simulink model "CondenserMic"  (R2024a)
settings: Solver=daessc  StartTime=0.0  StopTime=T  MaxStep=1e-4  RelTol=1e-3
PreLoadFcn:
  | f_in = 1000;
model workspace (MAT data in the model file):
  A = Simulink.Parameter
  A.Value = Simulink.data.Expression
  A.Value.ExpressionString = "pi*r^2"
  A.Complexity = 'real'
  A.Dimensions = -1
  A.Description = 'diaphragm area'
  A.DataType = 'auto'
  A.DocUnits = 'm^2'
  A_bp = Simulink.Parameter
  A_bp.Value = Simulink.data.Expression
  A_bp.Value.ExpressionString = "pi*r_bp^2"
  A_bp.Complexity = 'real'
  A_bp.Dimensions = -1
  A_bp.DataType = 'auto'
  A_bp.DocUnits = 'm^2'
  Ceo = Simulink.Parameter
  Ceo.Value = 1.85e-11
  Ceo.Complexity = 'real'
  Ceo.Dimensions = [1 1]
  Ceo.Description = 'microphone open circuit capacitance'
  Ceo.DataType = 'auto'
  Ceo.DocUnits = 'F'
  N_hole = Simulink.Parameter
  N_hole.Value = 6
  N_hole.Complexity = 'real'
  N_hole.Dimensions = [1 1]
  N_hole.Description = 'number of holes on back plate'
  N_hole.DataType = 'auto'
  N_vent = Simulink.Parameter
  N_vent.Value = 6
  N_vent.Complexity = 'real'
  N_vent.Dimensions = [1 1]
  N_vent.Description = 'number of rear vent'
  N_vent.DataType = 'auto'
  T = Simulink.Parameter
  T.Value = 5
  T.Complexity = 'real'
  T.Dimensions = [1 1]
  T.Description = 'simulation time '
  T.DataType = 'auto'
  Vb = Simulink.Parameter
  Vb.Value = 1.264e-07
  Vb.Complexity = 'real'
  Vb.Dimensions = [1 1]
  Vb.Description = 'rear cavity volume'
  Vb.DataType = 'auto'
  Vb.DocUnits = 'm^3'
  c = Simulink.Parameter
  c.Value = 343
  c.Complexity = 'real'
  c.Dimensions = [1 1]
  c.Description = 'sound speed in air'
  c.DataType = 'auto'
  c.DocUnits = 'm/s'
  d1 = Simulink.Parameter
  d1.Value = 0.002032
  d1.Complexity = 'real'
  d1.Dimensions = [1 1]
  d1.Description = 'Radius of the circle intersecting the holes'
  d1.DataType = 'auto'
  d1.DocUnits = 'm'
  dt = Simulink.Parameter
  dt.Value = 2.08333333333e-05
  dt.Complexity = 'real'
  dt.Dimensions = [1 1]
  dt.Description = 'sample time'
  dt.DataType = 'auto'
  eps0 = Simulink.Parameter
  eps0.Value = 8.85e-12
  eps0.Complexity = 'real'
  eps0.Dimensions = [1 1]
  eps0.Description = 'permittivity in vaicuum'
  eps0.DataType = 'auto'
  eps0.DocUnits = 'F/m'
  h_gap = Simulink.Parameter
  h_gap.Value = 2.077e-05
  h_gap.Complexity = 'real'
  h_gap.Dimensions = [1 1]
  h_gap.Description = 'air gap thickness '
  h_gap.DataType = 'auto'
  h_gap.DocUnits = 'm'
  h_hole = Simulink.Parameter
  h_hole.Value = 0.000843
  h_hole.Complexity = 'real'
  h_hole.Dimensions = [1 1]
  h_hole.Description = 'back plate holes depth (thickness)'
  h_hole.DataType = 'auto'
  h_hole.DocUnits = 'm'
  h_slot = Simulink.Parameter
  h_slot.Value = 0.0003048
  h_slot.Complexity = 'real'
  h_slot.Dimensions = [1 1]
  h_slot.Description = 'slot depth (thickness)'
  h_slot.DataType = 'auto'
  h_slot.DocUnits = 'm'
  h_vent = Simulink.Parameter
  h_vent.Value = 0.0015
  h_vent.Complexity = 'real'
  h_vent.Dimensions = [1 1]
  h_vent.Description = 'rear vent depth (thickness)'
  h_vent.DataType = 'auto'
  h_vent.DocUnits = 'm'
  l_slot = Simulink.Parameter
  l_slot.Value = Simulink.data.Expression
  l_slot.Value.ExpressionString = "2*pi*r"
  l_slot.Complexity = 'real'
  l_slot.Dimensions = -1
  l_slot.DataType = 'auto'
  l_slot.DocUnits = 'm'
  l_vent = Simulink.Parameter
  l_vent.Value = 0.00034
  l_vent.Complexity = 'real'
  l_vent.Dimensions = [1 1]
  l_vent.Description = 'rear vent length'
  l_vent.DataType = 'auto'
  l_vent.DocUnits = 'm'
  r = Simulink.Parameter
  r.Value = 0.00445
  r.Complexity = 'real'
  r.Dimensions = [1 1]
  r.Description = 'diaphragm radius'
  r.DataType = 'auto'
  r.DocUnits = 'm'
  r_bp = Simulink.Parameter
  r_bp.Value = 0.00361
  r_bp.Complexity = 'real'
  r_bp.Dimensions = [1 1]
  r_bp.Description = 'back plate radius'
  r_bp.DataType = 'auto'
  r_bp.DocUnits = 'm'
  r_hole = Simulink.Parameter
  r_hole.Value = 0.000508
  r_hole.Complexity = 'real'
  r_hole.Dimensions = [1 1]
  r_hole.Description = 'back plate holes radius'
  r_hole.DataType = 'auto'
  r_hole.DocUnits = 'm'
  rho = Simulink.Parameter
  rho.Value = 1.21
  rho.Complexity = 'real'
  rho.Dimensions = [1 1]
  rho.Description = 'air density'
  rho.DataType = 'auto'
  rho.DocUnits = 'kg/m^3'
  w_slot = Simulink.Parameter
  w_slot.Value = 0.000838
  w_slot.Complexity = 'real'
  w_slot.Dimensions = [1 1]
  w_slot.Description = 'slot width'
  w_slot.DataType = 'auto'
  w_slot.DocUnits = 'm'
  w_vent = Simulink.Parameter
  w_vent.Value = 1.1e-05
  w_vent.Complexity = 'real'
  w_vent.Dimensions = [1 1]
  w_vent.Description = 'rear vent width'
  w_vent.DataType = 'auto'
  w_vent.DocUnits = 'm'
libraries: fl_lib x11, acoustic_lib x7, nesl_utility x3, ee_lib x1
settings Model: Creator=andychen  LastModifiedBy=jibrahim
settings DataIOCC: OutputOption=SpecifiedOutputTimes  OutputTimes=0:dt:T  Refine=0:5e-5:10

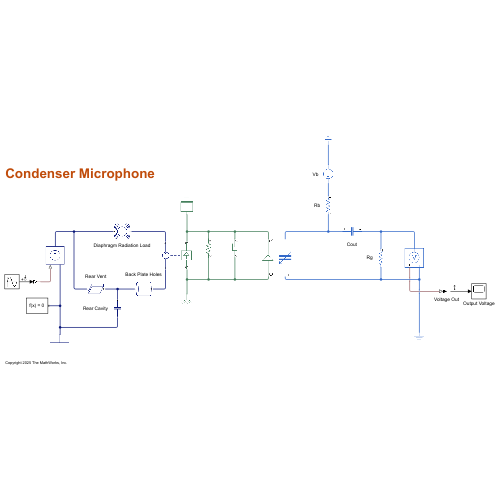
[thumbnail: Simulink's stored preview of the top-level diagram]
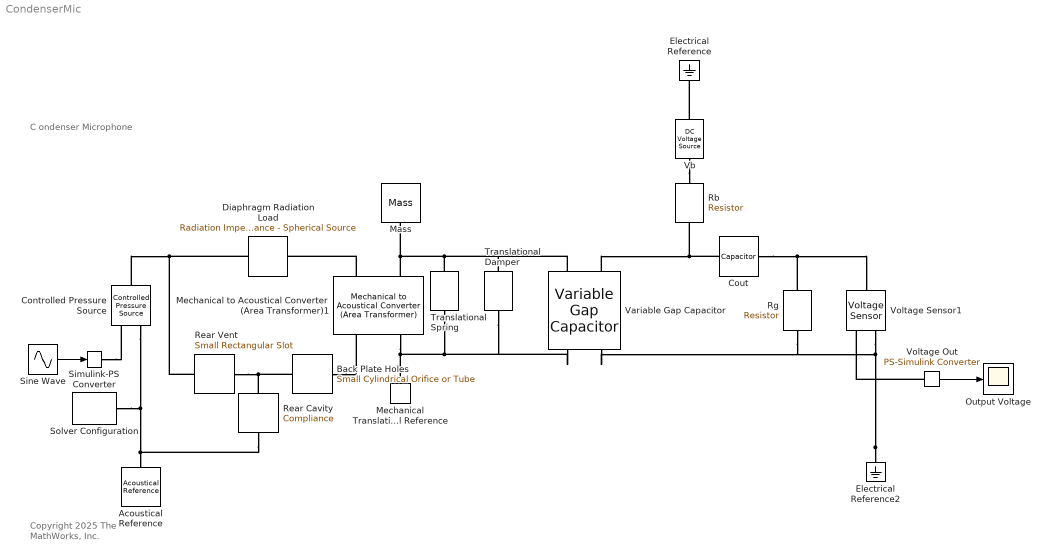
== system CondenserMic ==
  note: C ondenser Microphone
  note: Copyright 2025 The MathWorks, Inc.
  Acoustical Reference : acoustic_lib/Acoustical Elements/Acoustical Reference
      settings: SourceProductName=Acoustic  InternalSimscapePortConfiguration="{\"Bottom\":[],\"Left\":[{\"id\":\"pp\",\"label\":\"\",\"type\":\"acoustic.acoustic\"}],\"Right\":[],\"Top\":[]}"
  Back Plate Holes : acoustic_lib/Applications/Tubes and Horns/Small Cylindrical Orifice or Tube  l=h_hole m  r=r_hole m  N=N_hole
      settings: SourceProductName=Acoustic  InternalSimscapePortConfiguration="{\"Bottom\":[],\"Left\":[{\"id\":\"pa\",\"label\":\"+\",\"type\":\"acoustic.acoustic\"}],\"Right\":[{\"id\":\"na\",\"label\":\"-\",\"type\":\"acoustic.acoustic\"}],\"Top\":[]}"
  Controlled Pressure Source : acoustic_lib/Acoustical Sources/Controlled Pressure Source
      settings: SourceProductName=Acoustic  InternalSimscapePortConfiguration="{\"Bottom\":[],\"Left\":[{\"id\":\"pp\",\"label\":\"\",\"type\":\"acoustic.acoustic\"}],\"Right\":[{\"id\":\"pT\",\"label\":\"\",\"type\":\"input\"},{\"id\":\"nn\",\"label\":\"\",\"type\":\"acoustic.acoustic\"}],\"Top\":[]}"
  Cout : fl_lib/Electrical/Electrical Elements/Capacitor  c=1e-12 F  r=1e-6 Ohm  g=0 1/Ohm  i_specify=off  i_priority=None  i=0 A  i_nominal_specify=off  i_nominal_value=1  i_nominal_unit=A  v_specify=off  v_priority=None  v=0 V  v_nominal_specify=off  v_nominal_value=1  v_nominal_unit=V  vc_specify=off  vc_priority=High  vc=0 V  vc_nominal_specify=off  vc_nominal_value=1  vc_nominal_unit=V
  Diaphragm Radiation Load : acoustic_lib/Radiation Impedance/Radiation Impedance - Spherical Source  r=r m
      settings: SourceProductName=Acoustic  InternalSimscapePortConfiguration="{\"Bottom\":[],\"Left\":[{\"id\":\"pa\",\"label\":\"+\",\"type\":\"acoustic.acoustic\"}],\"Right\":[{\"id\":\"na\",\"label\":\"-\",\"type\":\"acoustic.acoustic\"}],\"Top\":[]}"
  Electrical Reference : fl_lib/Electrical/Electrical Elements/Electrical Reference
  Electrical Reference2 : fl_lib/Electrical/Electrical Elements/Electrical Reference
  Mass : fl_lib/Mechanical/Translational Elements/Mass  mass=9.22e-7 kg  num_ports=foundation.enum.numPorts2.one  v_specify=off  v_priority=High  v=0 m/s  v_nominal_specify=off  v_nominal_value=1  v_nominal_unit=m/s  f_specify=off  f_priority=None  f=0 N  f_nominal_specify=off  f_nominal_value=1  f_nominal_unit=N
  Mechanical Translational Reference : fl_lib/Mechanical/Translational Elements/Mechanical Translational Reference
  Mechanical to Acoustical Converter (Area Transformer)1 : acoustic_lib/Transformers/Mechanical to Acoustical Converter (Area Transformer)  Sd=A m^2  u_specify=off  u_priority=None  u=0 m^3/s  u_nominal_specify=off  u_nominal_value=1  u_nominal_unit=m^3/s  p_specify=off  p_priority=None  p=0 Pa  p_nominal_specify=off  p_nominal_value=1  p_nominal_unit=Pa  f_specify=off  f_priority=None  f=0 N  f_nominal_specify=off  f_nominal_value=1  f_nominal_unit=N  v_specify=off  v_priority=None  v=0 m/s  v_nominal_specify=off  v_nominal_value=1  v_nominal_unit=m/s
      settings: SourceProductName=Acoustic  InternalSimscapePortConfiguration="{\"Bottom\":[],\"Left\":[{\"id\":\"pp\",\"label\":\"+\",\"type\":\"acoustic.acoustic\"},{\"id\":\"R\",\"label\":\"R\",\"type\":\"foundation.mechanical.translational.translational\"}],\"Right\":[{\"id\":\"nn\",\"label\":\"-\",\"type\":\"acoustic.acoustic\"},{\"id\":\"C\",\"label\":\"C\",\"type\":\"foundation.mechanical.translational.translational\"}],\"Top\":[]}"
  Output Voltage : Scope
  Rb : fl_lib/Electrical/Electrical Elements/Resistor  R=1e10 Ohm  i_specify=off  i_priority=None  i=0 A  i_nominal_specify=off  i_nominal_value=1  i_nominal_unit=A  v_specify=off  v_priority=None  v=0 V  v_nominal_specify=off  v_nominal_value=1  v_nominal_unit=V
  Rear Cavity : acoustic_lib/Acoustical Elements/Compliance  c=Vb/(rho*c^2) m^3/Pa  r_c=0 Pa*s/m^3  g_c=0 m^3/(Pa*s)  u_specify=off  u_priority=None  u=0 m^3/s  u_nominal_specify=off  u_nominal_value=1  u_nominal_unit=m^3/s  p_specify=off  p_priority=None  p=0 Pa  p_nominal_specify=off  p_nominal_value=1  p_nominal_unit=Pa  Pc_specify=off  Pc_priority=High  Pc=0 Pa  Pc_nominal_specify=off  Pc_nominal_value=1  Pc_nominal_unit=Pa
      settings: SourceProductName=Acoustic  InternalSimscapePortConfiguration="{\"Bottom\":[],\"Left\":[{\"id\":\"pp\",\"label\":\"+\",\"type\":\"acoustic.acoustic\"}],\"Right\":[{\"id\":\"nn\",\"label\":\"-\",\"type\":\"acoustic.acoustic\"}],\"Top\":[]}"
  Rear Vent : acoustic_lib/Applications/Tubes and Horns/Small Rectangular Slot  l=h_vent m  w=l_vent m  h=w_vent m  N=N_vent
      settings: SourceProductName=Acoustic  InternalSimscapePortConfiguration="{\"Bottom\":[],\"Left\":[{\"id\":\"pa\",\"label\":\"+\",\"type\":\"acoustic.acoustic\"}],\"Right\":[{\"id\":\"na\",\"label\":\"-\",\"type\":\"acoustic.acoustic\"}],\"Top\":[]}"
  Rg : fl_lib/Electrical/Electrical Elements/Resistor  R=1e11 Ohm  i_specify=off  i_priority=None  i=0 A  i_nominal_specify=off  i_nominal_value=1  i_nominal_unit=A  v_specify=off  v_priority=None  v=0 V  v_nominal_specify=off  v_nominal_value=1  v_nominal_unit=V
  Simulink-PS Converter : nesl_utility/Simulink-PS Converter  PhysicalDomain=network_engine_domain  SubClassName=ps_input  LeftPortType=input  RightPortType=output  PseudoPeriodic=off  Frequencies=[]  NoiseDistribution=none  NoiseParameters=[]  Unit=1  AffineConversion=off  FilteringAndDerivatives=provide  SimscapeFilterOrder=1  InputFilterTimeConstant=0.001  UdotUserProvided=0
  Sine Wave : Sin  Frequency=2*pi*f_in  SampleTime=0
  Solver Configuration : nesl_utility/Solver Configuration  PhysicalDomain=network_engine_domain  SubClassName=solver  LeftPortType=input  RightPortType=generic  Tones=[]  Harmonics=[]  SimulateNoise=off  Profile=off  UseLocalSampling=off  EnableSwitchedLinearOptims=on  FrequencyDomain=off  UseCCode=off  RelTol=0.001  AbsTol=0.001  MinStep=1e-09  ToWorkspace=off  RevertToSquareIcSolve=off  NumHomotopyIterations=100  PhasorMode=off  PhasorModeNumHarmonics=1  ConsistencySolver=NEWTON_XTOL_AFTER_FTOL  IndexReductionMethod=DerivativeReplacement  DoDC=off  ResidualTolerance=1e-09  ConsistencyTolSource=GLOBAL  ConsistencyAbsTol=0.001  ConsistencyRelTol=0.001  ConsistencyTolFactor=0.001  UseLocalSolver=off  LocalSolverChoice=NE_BACKWARD_EULER_ADVANCER  ResolveIndetEquations=on  FunctionEvalNumThread=1  LocalSolverSampleTime=0.001  DoFixedCost=off  MaxNonlinIter=3  MaxModeIter=2  ComputeImpulses=off  ImpulseIterations=2  LinearAlgebra=auto  LinearAlgebraNumThread=0  EquationFormulation=NE_TIME_EF  DelaysMemoryBudget=1024  AutomaticFiltering=on  FilteringTimeConstant=0.001  PartitionStorageMethod=AS_NEEDED  PartitionMemoryBudget=1024  PartitionMethod=ROBUST  MultibodyUseLocalSolver=off  MultibodyLocalSolverChoice=ODE1  MultibodyLocalSolverSampleTime=0.001
  Translational Damper : fl_lib/Mechanical/Translational Elements/Translational Damper  D=0.4 N*s/m  v_specify=off  v_priority=None  v=0 m/s  v_nominal_specify=off  v_nominal_value=1  v_nominal_unit=m/s  f_specify=off  f_priority=None  f=0 N  f_nominal_specify=off  f_nominal_value=1  f_nominal_unit=N
  Translational Spring : fl_lib/Mechanical/Translational Elements/Translational Spring  spr_rate=4.4e4 N/m  v_specify=off  v_priority=None  v=0 m/s  v_nominal_specify=off  v_nominal_value=1  v_nominal_unit=m/s  f_specify=off  f_priority=None  f=0 N  f_nominal_specify=off  f_nominal_value=1  f_nominal_unit=N  x_specify=off  x_priority=High  x=0 m  x_nominal_specify=off  x_nominal_value=1  x_nominal_unit=m
  Variable Gap Capacitor : ee_lib/Passive/Variable Gap Capacitor  A=A_bp m^2  d=h_gap m  ModelElasticDielectric=false  epsr=1.0  E=0 Pa  v_specify=off  v_priority=None  v=0 V  v_nominal_specify=off  v_nominal_value=1  v_nominal_unit=V  i_specify=off  i_priority=None  i=0 A  i_nominal_specify=off  i_nominal_value=1  i_nominal_unit=A  Q_specify=off  Q_priority=High  Q=0 C  Q_nominal_specify=off  Q_nominal_value=1  Q_nominal_unit=C  u_specify=off  u_priority=None  u=0 m/s  u_nominal_specify=off  u_nominal_value=1  u_nominal_unit=m/s  f_specify=off  f_priority=None  f=0 N  f_nominal_specify=off  f_nominal_value=1  f_nominal_unit=N  x_specify=off  x_priority=High  x=0 m  x_nominal_specify=off  x_nominal_value=1  x_nominal_unit=m
      settings: InternalSimscapePortConfiguration="{\"Bottom\":[],\"Left\":[{\"id\":\"p\",\"label\":\"+\",\"type\":\"foundation.electrical.electrical\"},{\"id\":\"R\",\"label\":\"R\",\"type\":\"foundation.mechanical.translational.translational\"}],\"Right\":[{\"id\":\"n\",\"label\":\"-\",\"type\":\"foundation.electrical.electrical\"},{\"id\":\"C\",\"label\":\"C\",\"type\":\"foundation.mechanical.translational.translational\"}],\"Top\":[]}"
  Vb : fl_lib/Electrical/Electrical Sources/DC Voltage Source  v0=200 V
  Voltage Out : nesl_utility/PS-Simulink Converter  PhysicalDomain=network_engine_domain  SubClassName=ps_output  LeftPortType=input  RightPortType=output  PseudoPeriodic=off  Frequencies=[]  VectorFormat=inherit  Unit=inherit  AffineConversion=off
  Voltage Sensor1 : fl_lib/Electrical/Electrical Sensors/Voltage Sensor
  wires:
  Voltage Out/1 -> Output Voltage/1
  Sine Wave/1 -> Simulink-PS Converter/1
  connections:
  Variable Gap Capacitor/LConn2 -- Translational Damper/LConn1 -- Translational Spring/LConn1 -- Mechanical to Acoustical Converter (Area Transformer)1/LConn2 -- Mass/LConn1
  Mechanical Translational Reference/LConn1 -- Mechanical to Acoustical Converter (Area Transformer)1/RConn2 -- Variable Gap Capacitor/RConn2 -- Translational Damper/RConn1 -- Translational Spring/RConn1
  Vb/RConn1 -- Electrical Reference/LConn1
  Vb/LConn1 -- Rb/LConn1
  Voltage Out/LConn1 -- Voltage Sensor1/RConn1
  Simulink-PS Converter/RConn1 -- Controlled Pressure Source/RConn1
  Rg/LConn1 -- Cout/RConn1 -- Voltage Sensor1/LConn1
  Rear Cavity/LConn1 -- Rear Vent/LConn1 -- Back Plate Holes/RConn1
  Diaphragm Radiation Load/LConn1 -- Controlled Pressure Source/LConn1 -- Rear Vent/RConn1
  Cout/LConn1 -- Variable Gap Capacitor/LConn1 -- Rb/RConn1
  Solver Configuration/RConn1 -- Rear Cavity/RConn1 -- Acoustical Reference/LConn1 -- Controlled Pressure Source/RConn2
  Back Plate Holes/LConn1 -- Mechanical to Acoustical Converter (Area Transformer)1/RConn1
  Electrical Reference2/LConn1 -- Variable Gap Capacitor/RConn1 -- Rg/RConn1 -- Voltage Sensor1/RConn2
  Mechanical to Acoustical Converter (Area Transformer)1/LConn1 -- Diaphragm Radiation Load/RConn1
